simulink model "KalmanFilterTest"  (R2018b)
settings: Solver=VariableStepAuto  StartTime=0.0  StopTime=Tf  RelTol=1e-5
values from neighbouring files (symbols this model uses):
  A = [0 1;2 -1]    [KirkFHLQR.m]    (also in tvkalman1by1Constant.m = evalt(A,Time); tvkalman1by1LTV.m = tvmat(Adata,t); tvkalman2by2WithSL.m = [A1 -1;-2 A2])
  B = [0; 1]    [KirkFHLQR.m]    (also in tvkalman1by1Constant.m = 1; tvkalman1by1LTV.m = 1; tvkalman2by2WithSL.m = [1;1])
  Bw = 1    [tvkalman1by1LTV.m]    (also in tvkalman2by2WithSL.m = [1;1])
  C = eye(2)    [KirkFHLQR.m]    (also in tvkalman1by1Constant.m = 1; tvkalman1by1LTV.m = 1; tvkalman2by2WithSL.m)
  D = 0    [KirkFHLQR.m]    (also in tvkalman1by1Constant.m; tvkalman1by1LTV.m; tvkalman2by2WithSL.m = [0;0])
  Dw = 0    [tvkalman1by1LTV.m]    (also in tvkalman2by2WithSL.m = [0;0])
undefined symbols (not defined in the file or in its folder): Lfh
libraries: ltvlib x5
settings Model: Creator=jyotbuch  LastModifiedBy=jyotbuch

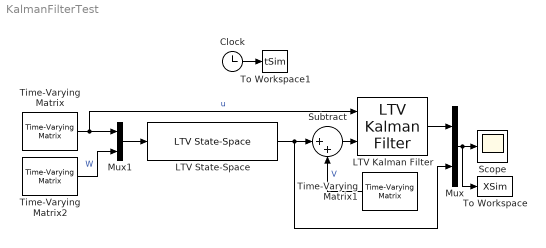
== system KalmanFilterTest ==
  Clock : Clock
  LTV Kalman Filter : ltvlib/LTV Kalman Filter  A=A  B=B  C=C  D=D  xhat0=xhat0  L=Lfh
      settings: SourceProductName=Linear Time-Varying Systems Toolbox
  LTV State-Space : ltvlib/LTV State-Space  A=A  B=[B Bw]  C=C  D=[D Dw]  x0=x0
      settings: SourceProductName=Linear Time-Varying Systems Toolbox
  Mux : Mux  Inputs=2
  Mux1 : Mux  Inputs=2
  Scope : Scope
  Subtract : Sum  Inputs=|++
  Time-Varying Matrix : ltvlib/Time-Varying Matrix  M=u  vec1D=on
      settings: SourceProductName=Linear Time-Varying Systems Toolbox
  Time-Varying Matrix1 : ltvlib/Time-Varying Matrix  M=V  vec1D=on
      settings: SourceProductName=Linear Time-Varying Systems Toolbox
  Time-Varying Matrix2 : ltvlib/Time-Varying Matrix  M=W  vec1D=on
      settings: SourceProductName=Linear Time-Varying Systems Toolbox
  To Workspace : ToWorkspace  VariableName=XSim  SampleTime=-1
  To Workspace1 : ToWorkspace  VariableName=tSim  SampleTime=-1
  wires:
  Time-Varying Matrix/1 -> Mux1/1, LTV Kalman Filter/1  "u"
  LTV State-Space/1 -> Mux/2, Subtract/1
  Subtract/1 -> LTV Kalman Filter/2
  Time-Varying Matrix1/1 -> Subtract/2  "V"
  Mux/1 -> To Workspace/1, Scope/1
  LTV Kalman Filter/1 -> Mux/1
  Clock/1 -> To Workspace1/1
  Mux1/1 -> LTV State-Space/1
  Time-Varying Matrix2/1 -> Mux1/2  "W"
